simulink model "modelingusingsimulink"  (R2023a)
settings: Solver=VariableStepAuto  StartTime=0.0  StopTime=10.0  RelTol=1e-3
undefined symbols (not defined in the file): Eact, F, K, R
settings Model: Creator=meghn  LastModifiedBy=meghn

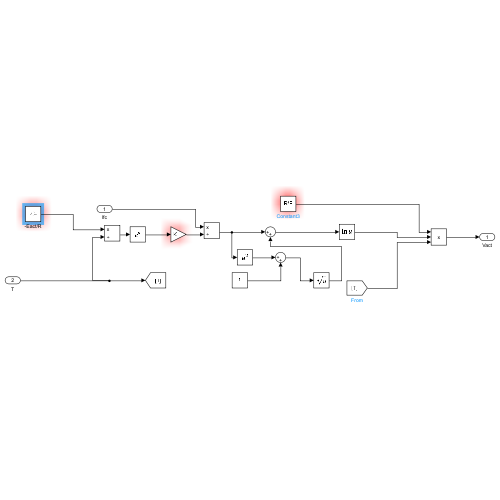
[thumbnail: Simulink's stored preview of the top-level diagram]
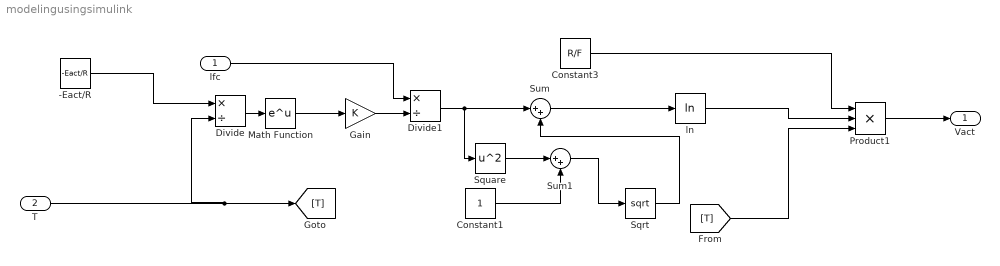
== system modelingusingsimulink ==
  lfc : Inport
  T : Inport  Port=2
  -Eact/R : Constant  Value=-Eact/R
  Constant1 : Constant
  Constant3 : Constant  Value=R/F
  Divide : Product  Inputs=*/
  Divide1 : Product  Inputs=*/
  Gain : Gain  Gain=K
  Math Function : Math
  Product1 : Product  Inputs=3
  Sqrt : Sqrt
  Square : Math  Operator=square
  Sum : Sum  Inputs=|++
  Sum1 : Sum  Inputs=|++
  ln : Math  Operator=log
  Vact : Outport
  wires:
  -Eact/R/1 -> Divide/1
  T/1 -> Divide/2, [T]
  Divide/1 -> Math Function/1
  Math Function/1 -> Gain/1
  lfc/1 -> Divide1/1
  Gain/1 -> Divide1/2
  Divide1/1 -> Square/1, Sum/1
  Square/1 -> Sum1/1
  Constant1/1 -> Sum1/2
  Sum1/1 -> Sqrt/1
  Sqrt/1 -> Sum/2
  Sum/1 -> ln/1
  ln/1 -> Product1/2
  Constant3/1 -> Product1/1
  [T] -> Product1/3
  Product1/1 -> Vact/1
